simulink model "BE_mecatronique_4"  (R2022b)
settings: Solver=VariableStepAuto  StartTime=0.0  StopTime=100  RelTol=1e-3
values from neighbouring files (symbols this model uses):
  assist = 2    [BE_eletr.m]
  Jt = M*Rw^2    (= 10.0188)    [BE_eletr.m]
  lambm = 0.0744    [BE_eletr.m]
  Ls = 0.0021    [BE_eletr.m]
  Np = 52    [BE_eletr.m]
  Rs = 0.124    [BE_eletr.m]
  s = 0.07    [BE_eletr.m]
libraries: slpidlib x2
settings Model: Creator=antoi  LastModifiedBy=guilhermepifferchristo
settings SolverCC: AlgebraicLoopSolver=TrustRegion
settings DebuggingCC: AlgebraicLoopMsg=none  UnconnectedInputMsg=warning  UnconnectedOutputMsg=warning  UnconnectedLineMsg=warning  SFMachineParentedDataDiag=warning
settings ModelReferenceCC: EnableRefExpFcnMdlSchedulingChecks=on

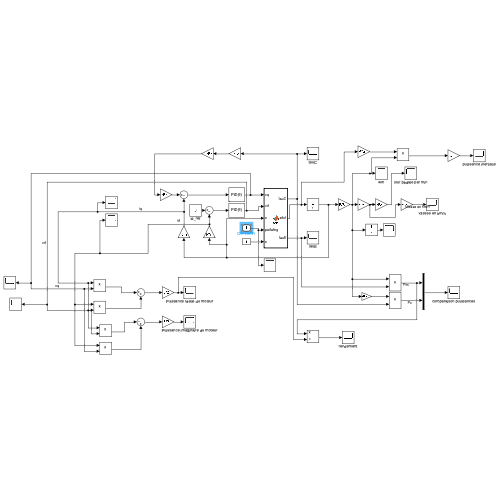
[thumbnail: Simulink's stored preview of the top-level diagram]
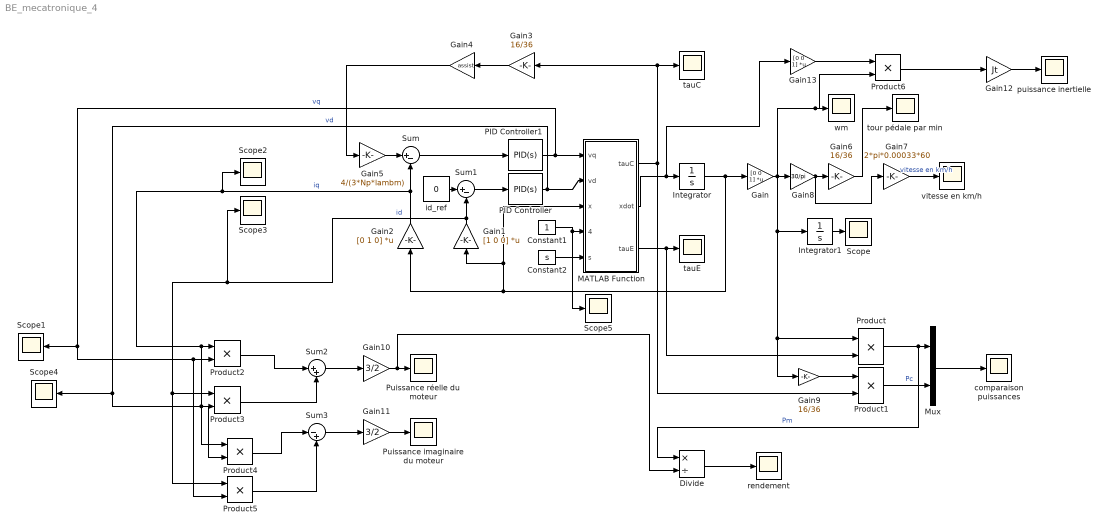
== system BE_mecatronique_4 ==
  Constant1 : Constant
  Constant2 : Constant  Value=s
  Divide : Product  Inputs=*/
  Gain : Gain  Gain=[0 0 1]  Multiplication=Matrix(K*u)
  Gain1 : Gain  Gain=[1 0 0]  Multiplication=Matrix(K*u)
  Gain10 : Gain  Gain=3/2
  Gain11 : Gain  Gain=3/2
  Gain12 : Gain  Gain=Jt
  Gain13 : Gain  Gain=[0 0 1]  Multiplication=Matrix(K*u)
  Gain2 : Gain  Gain=[0 1 0]  Multiplication=Matrix(K*u)
  Gain3 : Gain  Gain=16/36
  Gain4 : Gain  Gain=assist
  Gain5 : Gain  Gain=4/(3*Np*lambm)
  Gain6 : Gain  Gain=16/36
  Gain7 : Gain  Gain=2*pi*0.00033*60
  Gain8 : Gain  Gain=30/pi
  Gain9 : Gain  Gain=16/36
  Integrator : Integrator  InitialCondition=[0 ;0 ;0]
  Integrator1 : Integrator
  MATLAB Function : MATLAB Function  TreatAsAtomicUnit=on
  Mux : Mux  Inputs=2
  PID Controller : slpidlib/PID Controller  Controller=PID  Form=Parallel  TimeDomain=Continuous-time  UseExternalTs=off  SampleTime=-1  IntegratorMethod=Forward Euler  FilterMethod=Forward Euler  ControllerParametersSource=internal  P=Rs  I=Rs*Rs/Ls  UseKiTs=off  D=0  N=100  UseFilter=on  TunerSelectOption=Transfer Function Based (PID Tuner App)  InitialConditionSource=internal  InitialConditionForIntegrator=0  InitialConditionForFilter=0  DifferentiatorICPrevScaledInput=0  ExternalReset=none  TrackingMode=off  Kt=1  LimitOutput=off  SatLimitsSource=internal  UpperSaturationLimit=inf  LowerSaturationLimit=-inf  LinearizeAsGain=on  AntiWindupMode=none  Kb=1  LimitIntegrator=off  UpperIntegratorSaturationLimit=inf  LowerIntegratorSaturationLimit=-inf  POutMin=[]  POutMax=[]  IOutMin=[]  IOutMax=[]  DOutMin=[]  DOutMax=[]  NOutMin=[]  NOutMax=[]  SumOutMin=[]  SumOutMax=[]  SaturationOutMin=[]  SaturationOutMax=[]  PParamMin=[]  PParamMax=[]  IParamMin=[]  IParamMax=[]  DParamMin=[]  DParamMax=[]  NParamMin=[]  NParamMax=[]  KbParamMin=[]  KbParamMax=[]  KtParamMin=[]  KtParamMax=[]  KbOutMin=[]  KbOutMax=[]  KtOutMin=[]  KtOutMax=[]  IntegratorOutMin=[]  IntegratorOutMax=[]  FilterOutMin=[]  FilterOutMax=[]  SumI1OutMin=[]  SumI1OutMax=[]  SumI2OutMin=[]  SumI2OutMax=[]  SumI3OutMin=[]  SumI3OutMax=[]  SumI4OutMin=[]  SumI4OutMax=[]  SumDOutMin=[]  SumDOutMax=[]  DifferentiatorOutMin=[]  DifferentiatorOutMax=[]  FilterDiffOutCoefMin=[]  FilterDiffOutCoefMax=[]  ReciprocalOutMin=[]  ReciprocalOutMax=[]  SumDenOutMin=[]  SumDenOutMax=[]  SumNumOutMin=[]  SumNumOutMax=[]  DivideOutMin=[]  DivideOutMax=[]  UdiffTsProdOutMin=[]  UdiffTsProdOutMax=[]  NTsProdOutMin=[]  NTsProdOutMax=[]  UintegralTsProdOutMin=[]  UintegralTsProdOutMax=[]  UngainTsProdOutMin=[]  UngainTsProdOutMax=[]  ClampingZeroOutDataTypeStr=Inherit: Inherit via back propagation  ClampingZeroOutMin=[]  ClampingZeroOutMax=[]  FilterDenConstantOutDataTypeStr=Inherit: Inherit via back propagation  FilterDenConstantOutMin=[]  FilterDenConstantOutMax=[]  PCopyOutDataTypeStr=Inherit: Inherit via back propagation  PCopyOutMin=[]  PCopyOutMax=[]  NCopyOutDataTypeStr=Inherit: Inherit via back propagation  NCopyOutMin=[]  NCopyOutMax=[]  IntegratorContinuousStateAttributes=''  IntegratorStateMustResolveToSignalObject=off  IntegratorRTWStateStorageClass=Auto  FilterContinuousStateAttributes=''  FilterStateMustResolveToSignalObject=off  FilterRTWStateStorageClass=Auto  ParallelPVariant=InternalParameters  IdealPVariant=Disabled  IVariant=InternalParameters  DVariant=InternalParameters  IntegratorVariant=Continuous  SatVariant=Disabled  AWVariant=Passthrough  PCopyVariant=Disabled  TRVariant=Disabled  FdbkBlocksVariant=Forward  IdealPFdbkVariant=Disabled  SatFdbkVariant=Disabled  DerivativeFilterVariant=ContFilter  NVariant=InternalParameters  NCopyVariant=Disabled  FilterICVariant=InternalICsFilter  IntegratorICVariant=InternalICs  ExternalResetVariant=Disabled  TRSumVariant=Passthrough  SumFdbkVariant=Disabled  SumVariant=Sum_PID  TsampFilterVariant=InternalTs  TsampNgainVariant=Passthrough  TsampIntegralVariant=Passthrough  ExternalSaturationOutDataTypeStr=Inherit: Same as second input
  PID Controller1 : slpidlib/PID Controller  Controller=PID  Form=Parallel  TimeDomain=Continuous-time  UseExternalTs=off  SampleTime=-1  IntegratorMethod=Forward Euler  FilterMethod=Forward Euler  ControllerParametersSource=internal  P=Rs  I=Rs*Rs/Ls  UseKiTs=off  D=0  N=100  UseFilter=on  TunerSelectOption=Transfer Function Based (PID Tuner App)  InitialConditionSource=internal  InitialConditionForIntegrator=0  InitialConditionForFilter=0  DifferentiatorICPrevScaledInput=0  ExternalReset=none  TrackingMode=off  Kt=1  LimitOutput=off  SatLimitsSource=internal  UpperSaturationLimit=inf  LowerSaturationLimit=-inf  LinearizeAsGain=on  AntiWindupMode=none  Kb=1  LimitIntegrator=off  UpperIntegratorSaturationLimit=inf  LowerIntegratorSaturationLimit=-inf  POutMin=[]  POutMax=[]  IOutMin=[]  IOutMax=[]  DOutMin=[]  DOutMax=[]  NOutMin=[]  NOutMax=[]  SumOutMin=[]  SumOutMax=[]  SaturationOutMin=[]  SaturationOutMax=[]  PParamMin=[]  PParamMax=[]  IParamMin=[]  IParamMax=[]  DParamMin=[]  DParamMax=[]  NParamMin=[]  NParamMax=[]  KbParamMin=[]  KbParamMax=[]  KtParamMin=[]  KtParamMax=[]  KbOutMin=[]  KbOutMax=[]  KtOutMin=[]  KtOutMax=[]  IntegratorOutMin=[]  IntegratorOutMax=[]  FilterOutMin=[]  FilterOutMax=[]  SumI1OutMin=[]  SumI1OutMax=[]  SumI2OutMin=[]  SumI2OutMax=[]  SumI3OutMin=[]  SumI3OutMax=[]  SumI4OutMin=[]  SumI4OutMax=[]  SumDOutMin=[]  SumDOutMax=[]  DifferentiatorOutMin=[]  DifferentiatorOutMax=[]  FilterDiffOutCoefMin=[]  FilterDiffOutCoefMax=[]  ReciprocalOutMin=[]  ReciprocalOutMax=[]  SumDenOutMin=[]  SumDenOutMax=[]  SumNumOutMin=[]  SumNumOutMax=[]  DivideOutMin=[]  DivideOutMax=[]  UdiffTsProdOutMin=[]  UdiffTsProdOutMax=[]  NTsProdOutMin=[]  NTsProdOutMax=[]  UintegralTsProdOutMin=[]  UintegralTsProdOutMax=[]  UngainTsProdOutMin=[]  UngainTsProdOutMax=[]  ClampingZeroOutDataTypeStr=Inherit: Inherit via back propagation  ClampingZeroOutMin=[]  ClampingZeroOutMax=[]  FilterDenConstantOutDataTypeStr=Inherit: Inherit via back propagation  FilterDenConstantOutMin=[]  FilterDenConstantOutMax=[]  PCopyOutDataTypeStr=Inherit: Inherit via back propagation  PCopyOutMin=[]  PCopyOutMax=[]  NCopyOutDataTypeStr=Inherit: Inherit via back propagation  NCopyOutMin=[]  NCopyOutMax=[]  IntegratorContinuousStateAttributes=''  IntegratorStateMustResolveToSignalObject=off  IntegratorRTWStateStorageClass=Auto  FilterContinuousStateAttributes=''  FilterStateMustResolveToSignalObject=off  FilterRTWStateStorageClass=Auto  ParallelPVariant=InternalParameters  IdealPVariant=Disabled  IVariant=InternalParameters  DVariant=InternalParameters  IntegratorVariant=Continuous  SatVariant=Disabled  AWVariant=Passthrough  PCopyVariant=Disabled  TRVariant=Disabled  FdbkBlocksVariant=Forward  IdealPFdbkVariant=Disabled  SatFdbkVariant=Disabled  DerivativeFilterVariant=ContFilter  NVariant=InternalParameters  NCopyVariant=Disabled  FilterICVariant=InternalICsFilter  IntegratorICVariant=InternalICs  ExternalResetVariant=Disabled  TRSumVariant=Passthrough  SumFdbkVariant=Disabled  SumVariant=Sum_PID  TsampFilterVariant=InternalTs  TsampNgainVariant=Passthrough  TsampIntegralVariant=Passthrough  ExternalSaturationOutDataTypeStr=Inherit: Same as second input
  Product{,1..6} (7 alike) : Product
  Puissance imaginaire du moteur : Scope
  Puissance réelle du moteur : Scope
  Scope{,1..5} (6 alike) : Scope
  Sum : Sum  Inputs=|+-
  Sum1 : Sum  Inputs=|+-
  Sum2 : Sum  Inputs=|++
  Sum3 : Sum  Inputs=|-+
  "comparaison puissances " : Scope
  id_ref : Constant  Value=0
  puissance inertielle : Scope
  rendement : Scope
  tauC : Scope
  tauE : Scope
  tour pédale par min : Scope
  vitesse en km/h : Scope
  wm : Scope
  wires:
  Integrator/1 -> Gain2/1, Gain1/1, MATLAB Function/3(x), Gain/1
  Integrator1/1 -> Scope/1
  MATLAB Function/2(xdot) -> Gain13/1, Integrator/1
  Gain/1 -> Gain9/1, Product/1, Integrator1/1, wm/1, Product6/2, Gain8/1
  id_ref/1 -> Sum1/1
  Sum1/1 -> PID Controller/1
  PID Controller/1 -> Scope4/1, Product4/2, Product3/2, MATLAB Function/2(vd)  "vd"
  PID Controller1/1 -> Product2/2, Product5/2, Scope1/1, MATLAB Function/1(vq)  "vq"
  Sum/1 -> PID Controller1/1
  Gain1/1 -> Scope3/1, Product3/1, Product5/1, Sum1/2  "id"
  Gain2/1 -> Scope2/1, Product4/1, Product2/1, Sum/2  "iq"
  Gain3/1 -> Gain4/1
  Gain5/1 -> Sum/1
  Gain4/1 -> Gain5/1
  Gain6/1 -> tour pédale par min/1
  Gain8/1 -> Gain7/1, Gain6/1
  Gain7/1 -> vitesse en km/h/1  "vitesse en km/h"
  Constant2/1 -> MATLAB Function/5(s)
  Mux/1 -> "comparaison puissances "/1
  Product/1 -> Divide/1, Mux/1  "Pm"
  Product1/1 -> Mux/2  "Pc"
  MATLAB Function/1(tauC) -> Product1/2, tauC/1, Gain3/1
  MATLAB Function/3(tauE) -> Product/2, tauE/1
  Gain9/1 -> Product1/1
  Product3/1 -> Sum2/2
  Product2/1 -> Sum2/1
  Gain10/1 -> Puissance réelle du moteur/1, Divide/2
  Sum2/1 -> Gain10/1
  Product4/1 -> Sum3/1
  Product5/1 -> Sum3/2
  Gain11/1 -> Puissance imaginaire du moteur/1
  Sum3/1 -> Gain11/1
  Divide/1 -> rendement/1
  Gain12/1 -> puissance inertielle/1
  Gain13/1 -> Product6/1
  Product6/1 -> Gain12/1
  Constant1/1 -> Scope5/1, MATLAB Function/4(pedaling)

== matlab function BE_mecatronique_4/MATLAB Function ==
  data: tauC output; vq input; vd input; xdot output; x input; tauE output; pedaling input; s input
function [tauC,xdot,tauE]= fcn(vq,vd,x,pedaling,s)
Rs = 0.124 ;
Ls = 0.0021 ;
Lambdam = 0.0744 ;
Np = 52 ;
M = 92 ;
Rw = 0.33 ;
Jt = M*Rw*Rw ;
Ca = 0.18 ;
g = 9.81 ;
tauE = (3*Np*Lambdam/4) * x(2) ;
tauC = (60 - (60/(4*pi))*x(3)*(16/36))*pedaling ; 
tauload = M*g*s*Rw + Ca*Rw*Rw*Rw*x(3)*x(3) ;
xdot1 =  -(Rs/Ls)*x(1) + (Np/2)*x(2)*x(3) + vd/Ls ;
xdot2 = -(Rs/Ls)*x(2) - (Np/2)*x(1)*x(3) - (Np/2)*(Lambdam/Ls)*x(3) + vq/Ls ; 
xdot3 = (1/Jt)*(tauE - tauload + tauC*16/36)  ;
xdot=[xdot1 ; xdot2 ; xdot3] ;
end
